simulink model "Wiper_Control_System"  (R2022a)
settings: Solver=FixedStepDiscrete  StartTime=0.0  StopTime=10.0  FixedStep=0.01  RelTol=1e-3
settings Model: DataDictionary=WCS_Data_Dictionary.sldd  EnableAccessToBaseWorkspace=off  DVExtractedSubsystem=Wiper_Control_System  Creator=jamesbond  LastModifiedBy=jamesbond
settings DebuggingCC: SignalRangeChecking=warning  FrameProcessingCompatibilityMsg=none
settings ConfigComp: DVMode=DesignErrorDetection  DVTestSuiteOptimization=Auto  DVDetectDeadLogic=on  DVDeadLogicObjectives=MCDC  DVDetectOutOfBounds=on  DVModelReferenceHarness=on  DVHarnessSource=Signal Editor

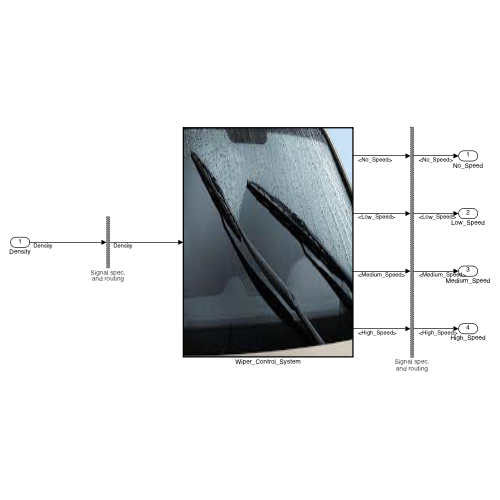
[thumbnail: Simulink's stored preview of the top-level diagram]
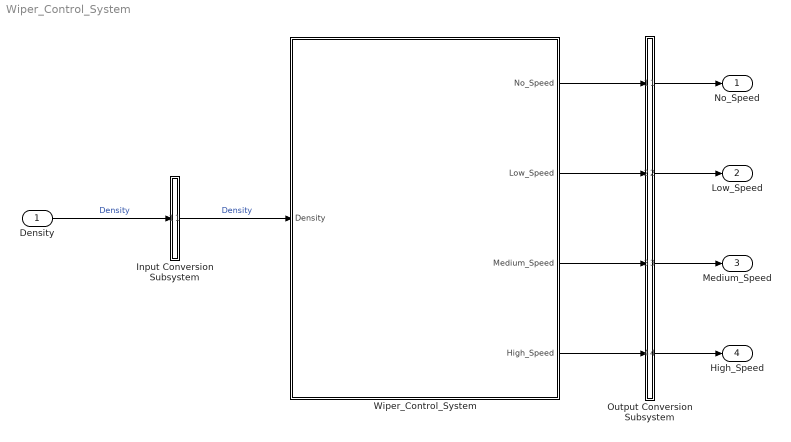
== system Wiper_Control_System ==
  Density : Inport  OutDataTypeStr=fixdt('ufix16_En4')  PortDimensions=[1]  SampleTime=[-1, 0]  Interpolate=off
  Input Conversion Subsystem : Subsystem  Tag=__SLT_ICS__  Description=|
      | Signal spec.
      | and routing
      settings: AttributesFormatString=%<Description>
  Output Conversion Subsystem : Subsystem  Tag=__SLT_OCS__  Description=|
      | Signal spec.
      | and routing
      settings: AttributesFormatString=%<Description>
  Wiper_Control_System : Subsystem  TreatAsAtomicUnit=on
      mask Display: image('$imagefile'); % Use "Edit Image" on toolstrip to change.
  No_Speed : Outport
  Low_Speed : Outport  Port=2
  Medium_Speed : Outport  Port=3
  High_Speed : Outport  Port=4
  wires:
  Density/1 -> Input Conversion Subsystem/1(Inport_1)  "Density"
  Output Conversion Subsystem/1(Outport_1) -> No_Speed/1
  Output Conversion Subsystem/2(Outport_2) -> Low_Speed/1
  Output Conversion Subsystem/3(Outport_3) -> Medium_Speed/1
  Output Conversion Subsystem/4(Outport_4) -> High_Speed/1
  Input Conversion Subsystem/1(Outport_1) -> Wiper_Control_System/1(Density)  "Density"
  Wiper_Control_System/1(No_Speed) -> Output Conversion Subsystem/1(Inport_1)
  Wiper_Control_System/2(Low_Speed) -> Output Conversion Subsystem/2(Inport_2)
  Wiper_Control_System/3(Medium_Speed) -> Output Conversion Subsystem/3(Inport_3)
  Wiper_Control_System/4(High_Speed) -> Output Conversion Subsystem/4(Inport_4)

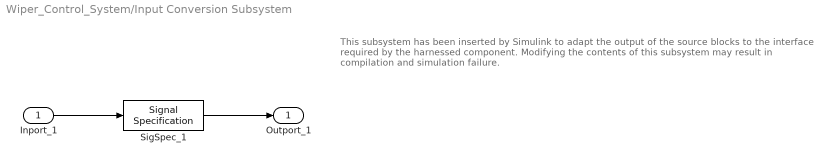
== system Wiper_Control_System/Input Conversion Subsystem ==
  note: This subsystem has been inserted by Simulink to adapt the output of the source blocks to the interface required by the harnessed component.
      |  Modifying the contents of this subsystem may result in compilation and simulation failure.
  Inport_1 : Inport
  SigSpec_1 : SignalSpecification  OutDataTypeStr=fixdt('ufix16_En4')  Dimensions=[1]  SampleTime=[-1, 0]
  Outport_1 : Outport
  wires:
  SigSpec_1/1 -> Outport_1/1
  Inport_1/1 -> SigSpec_1/1

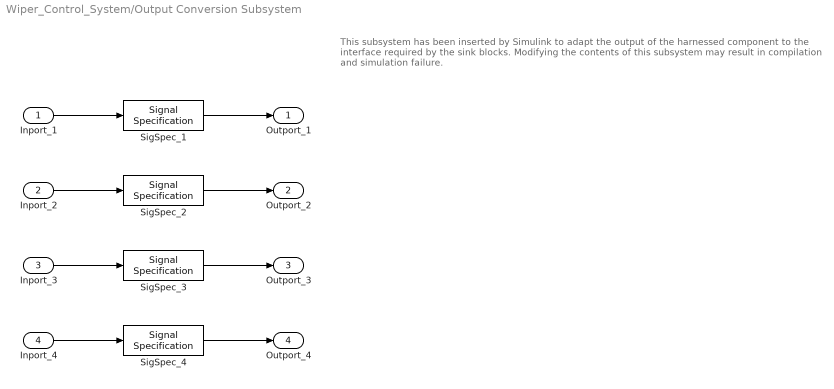
== system Wiper_Control_System/Output Conversion Subsystem ==
  note: This subsystem has been inserted by Simulink to adapt the output of the harnessed component to the interface required by the sink blocks.
      |  Modifying the contents of this subsystem may result in compilation and simulation failure.
  Inport_1 : Inport
  Inport_2 : Inport  Port=2
  Inport_3 : Inport  Port=3
  Inport_4 : Inport  Port=4
  SigSpec_1 : SignalSpecification  OutDataTypeStr=fixdt('sfix16_En4')  Dimensions=[1]
  SigSpec_2 : SignalSpecification  OutDataTypeStr=fixdt('ufix16_En9')  Dimensions=[1]
  SigSpec_3 : SignalSpecification  OutDataTypeStr=fixdt('sfix16_En4')  Dimensions=[1]
  SigSpec_4 : SignalSpecification  OutDataTypeStr=fixdt('sfix16_En4')  Dimensions=[1]
  Outport_1 : Outport
  Outport_2 : Outport  Port=2
  Outport_3 : Outport  Port=3
  Outport_4 : Outport  Port=4
  wires:
  Inport_1/1 -> SigSpec_1/1
  SigSpec_1/1 -> Outport_1/1
  Inport_2/1 -> SigSpec_2/1
  SigSpec_2/1 -> Outport_2/1
  Inport_3/1 -> SigSpec_3/1
  SigSpec_3/1 -> Outport_3/1
  Inport_4/1 -> SigSpec_4/1
  SigSpec_4/1 -> Outport_4/1

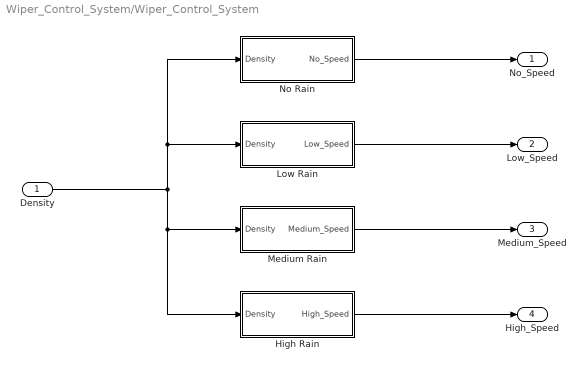
== system Wiper_Control_System/Wiper_Control_System ==
  Density : Inport  OutDataTypeStr=fixdt(0,16,4)
  High Rain : Subsystem
  Low Rain : Subsystem
  Medium Rain : Subsystem
  No Rain : Subsystem  TreatAsAtomicUnit=on
  No_Speed : Outport
  Low_Speed : Outport  Port=2
  Medium_Speed : Outport  Port=3
  High_Speed : Outport  Port=4
  wires:
  Density/1 -> No Rain/1(Density), Low Rain/1(Density), Medium Rain/1(Density), High Rain/1(Density)
  High Rain/1(High_Speed) -> High_Speed/1
  Medium Rain/1(Medium_Speed) -> Medium_Speed/1
  Low Rain/1(Low_Speed) -> Low_Speed/1
  No Rain/1(No_Speed) -> No_Speed/1

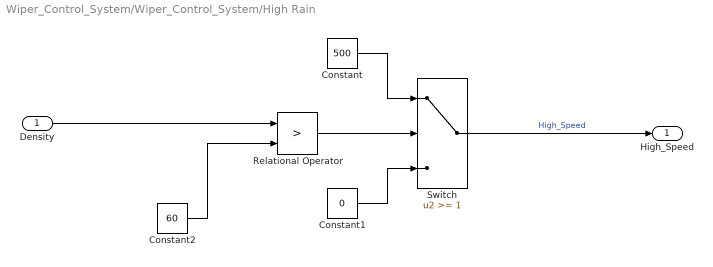
== system Wiper_Control_System/Wiper_Control_System/High Rain ==
  Density : Inport  OutDataTypeStr=fixdt(0,16, 4)
  Constant : Constant  Value=500  OutDataTypeStr=fixdt(0,16,7)
  Constant1 : Constant  Value=0  OutDataTypeStr=fixdt(1,16,4)
  Constant2 : Constant  Value=60  OutDataTypeStr=fixdt(0,16,10)
  Relational Operator : RelationalOperator  Operator=>  OutDataTypeStr=boolean  RndMeth=Simplest  InputSameDT=off
  Switch : Switch  Threshold=1  OutDataTypeStr=fixdt(1,16,4)  SaturateOnIntegerOverflow=off  InputSameDT=off
  High_Speed : Outport
  wires:
  Constant/1 -> Switch/1
  Constant1/1 -> Switch/3
  Constant2/1 -> Relational Operator/2
  Density/1 -> Relational Operator/1
  Relational Operator/1 -> Switch/2
  Switch/1 -> High_Speed/1  "High_Speed"

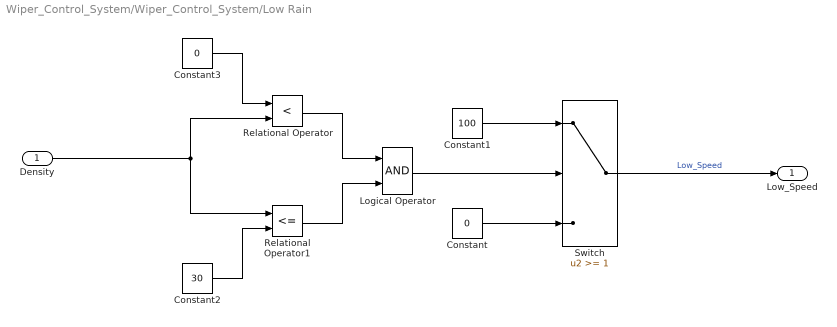
== system Wiper_Control_System/Wiper_Control_System/Low Rain ==
  Density : Inport  OutDataTypeStr=fixdt(0,16,4)
  Constant : Constant  Value=0  OutDataTypeStr=fixdt(1,16,4)
  Constant1 : Constant  Value=100  OutDataTypeStr=fixdt(0,16,9)
  Constant2 : Constant  Value=30  OutDataTypeStr=fixdt(0,16,11)
  Constant3 : Constant  Value=0  OutDataTypeStr=fixdt(1,16,4)
  Logical Operator : Logic  AllPortsSameDT=off  OutDataTypeStr=boolean
  Relational Operator : RelationalOperator  Operator=<  OutDataTypeStr=fixdt(1,16)  RndMeth=Simplest  InputSameDT=off
  Relational Operator1 : RelationalOperator  Operator=<=  OutDataTypeStr=boolean  RndMeth=Simplest  InputSameDT=off
  Switch : Switch  Threshold=1  OutDataTypeStr=fixdt(0,16,9)  SaturateOnIntegerOverflow=off  InputSameDT=off
  Low_Speed : Outport
  wires:
  Constant3/1 -> Relational Operator/1
  Density/1 -> Relational Operator1/1, Relational Operator/2
  Constant2/1 -> Relational Operator1/2
  Relational Operator1/1 -> Logical Operator/2
  Relational Operator/1 -> Logical Operator/1
  Constant/1 -> Switch/3
  Switch/1 -> Low_Speed/1  "Low_Speed"
  Constant1/1 -> Switch/1
  Logical Operator/1 -> Switch/2

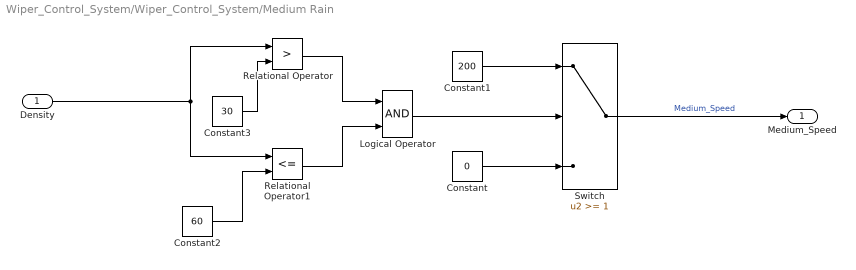
== system Wiper_Control_System/Wiper_Control_System/Medium Rain ==
  Density : Inport  OutDataTypeStr=fixdt(0,16,4)
  Constant : Constant  Value=0  OutDataTypeStr=fixdt(1,16,4)
  Constant1 : Constant  Value=200  OutDataTypeStr=fixdt(0,16,8)
  Constant2 : Constant  Value=60  OutDataTypeStr=fixdt(0,16,10)
  Constant3 : Constant  Value=30  OutDataTypeStr=fixdt(0,16,11)
  Logical Operator : Logic  AllPortsSameDT=off  OutDataTypeStr=boolean
  Relational Operator : RelationalOperator  Operator=>  OutDataTypeStr=boolean  RndMeth=Simplest  InputSameDT=off
  Relational Operator1 : RelationalOperator  Operator=<=  OutDataTypeStr=boolean  RndMeth=Simplest  InputSameDT=off
  Switch : Switch  Threshold=1  OutDataTypeStr=fixdt(1,16,4)  SaturateOnIntegerOverflow=off  InputSameDT=off
  Medium_Speed : Outport
  wires:
  Constant3/1 -> Relational Operator/2
  Switch/1 -> Medium_Speed/1  "Medium_Speed"
  Constant/1 -> Switch/3
  Constant1/1 -> Switch/1
  Logical Operator/1 -> Switch/2
  Constant2/1 -> Relational Operator1/2
  Relational Operator1/1 -> Logical Operator/2
  Density/1 -> Relational Operator1/1, Relational Operator/1
  Relational Operator/1 -> Logical Operator/1

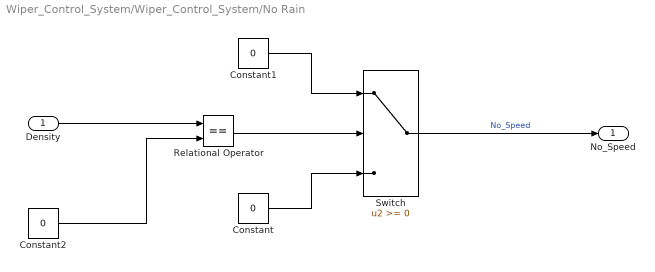
== system Wiper_Control_System/Wiper_Control_System/No Rain ==
  Density : Inport  OutDataTypeStr=fixdt(0,16,4)
  Constant : Constant  Value=0  OutDataTypeStr=fixdt(1,16,4)
  Constant1 : Constant  Value=0  OutDataTypeStr=fixdt(1,16,4)
  Constant2 : Constant  Value=0  OutDataTypeStr=fixdt(1,16,4)
  Relational Operator : RelationalOperator  Operator===  OutDataTypeStr=boolean  RndMeth=Simplest  InputSameDT=off
  Switch : Switch  OutDataTypeStr=fixdt(1,16,4)  SaturateOnIntegerOverflow=off  InputSameDT=off
  No_Speed : Outport
  wires:
  Density/1 -> Relational Operator/1
  Constant2/1 -> Relational Operator/2
  Constant1/1 -> Switch/1
  Constant/1 -> Switch/3
  Relational Operator/1 -> Switch/2
  Switch/1 -> No_Speed/1  "No_Speed"
